simulink model "only_rgb_image"  (R2019a)
settings: Solver=VariableStepAuto  StartTime=0.0  StopTime=10.0  RelTol=1e-3
undefined symbols (not defined in the file or in its folder): f
libraries: visiongeotforms x1, instrumentlib x1
settings Model: Creator=FJJ  LastModifiedBy=FJJ

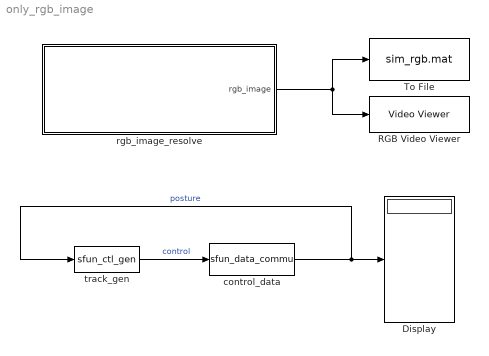
== system only_rgb_image ==
  Display : Display
  RGB Video Viewer : VideoViewer  FigPos=[818.6 719.6 724.8 428.8]
  To File : ToFile  Filename=sim_rgb.mat  MatrixName=rgb_image  SaveFormat=Timeseries
  control_data : S-Function  FunctionName=sfun_data_commu  Parameters='127.0.0.1', 59001, 2  SFunctionDeploymentMode=off  EnableBusSupport=off
  rgb_image_resolve : Subsystem
  track_gen : S-Function  FunctionName=sfun_ctl_gen  Parameters=-1  SFunctionDeploymentMode=off  EnableBusSupport=off
  wires:
  rgb_image_resolve/1(rgb_image) -> RGB Video Viewer/1, To File/1
  track_gen/1 -> control_data/1  "control"
  control_data/1 -> track_gen/1, Display/1  "posture"

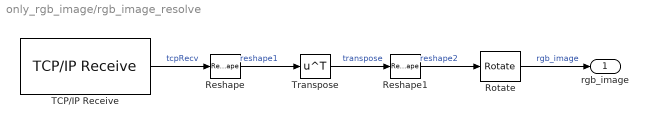
== system only_rgb_image/rgb_image_resolve ==
  Reshape : Reshape  OutputDimensionality=Customize  OutputDimensions=[3,307200]
  Reshape1 : Reshape  OutputDimensionality=Customize  OutputDimensions=[640,480,3]
  Rotate : visiongeotforms/Rotate  outSizeR=Expanded to fit rotated input image  src_angle=Specify via dialog  unit_angle=Degrees  angle=pi/2  maxAngle=pi  dispImage=Top-left corner  method=Table lookup  fillVal=0  interpMethod=Bilinear  roundingMode=Nearest  overflowMode=on  firstCoeffSlope=2^-10  prodOutputMode=Binary point scaling  prodOutputWordLength=32  prodOutputFracLength=10  prodOutputSlope=2^-10  accumSlope=2^-10  outputSlope=2^-10
      settings: SourceProductName=Computer Vision Toolbox
  TCP/IP Receive : instrumentlib/TCP//IP Receive  Host=127.0.0.1  Port=55555  DataSize=921600  EnableBlockingMode=on  Timeout=10  SampleTime=0.02  DataType=uint8  ByteOrder=BigEndian  ASCIIFormatting=%f,  Terminator=LF
      settings: SourceProductName=Instrument Control Toolbox
  Transpose : Math  Operator=transpose  SaturateOnIntegerOverflow=on
  rgb_image : Outport
  wires:
  Rotate/1 -> rgb_image/1  "rgb_image"
  Reshape/1 -> Transpose/1  "reshape1"
  Reshape1/1 -> Rotate/1  "reshape2"
  Transpose/1 -> Reshape1/1  "transpose"
  TCP/IP Receive/1 -> Reshape/1  "tcpRecv"
